simulink model "CONT_PID_CARRO"  (R2024b)
settings: Solver=VariableStepAuto  StartTime=0.0  StopTime=10.0  RelTol=1e-3
undefined symbols (not defined in the file): b_ta, K_tsa, K_tsia, T_s2
settings Model: Creator=juani  LastModifiedBy=juani

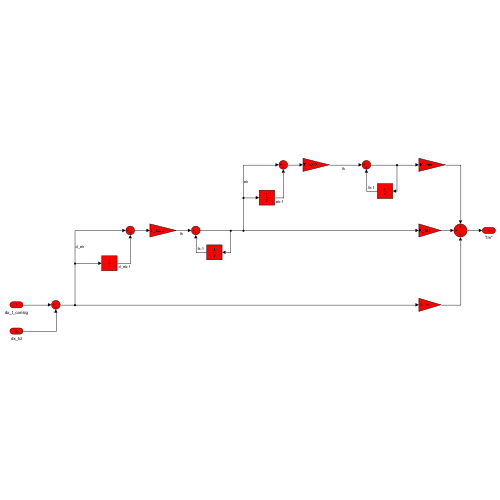
[thumbnail: Simulink's stored preview of the top-level diagram]
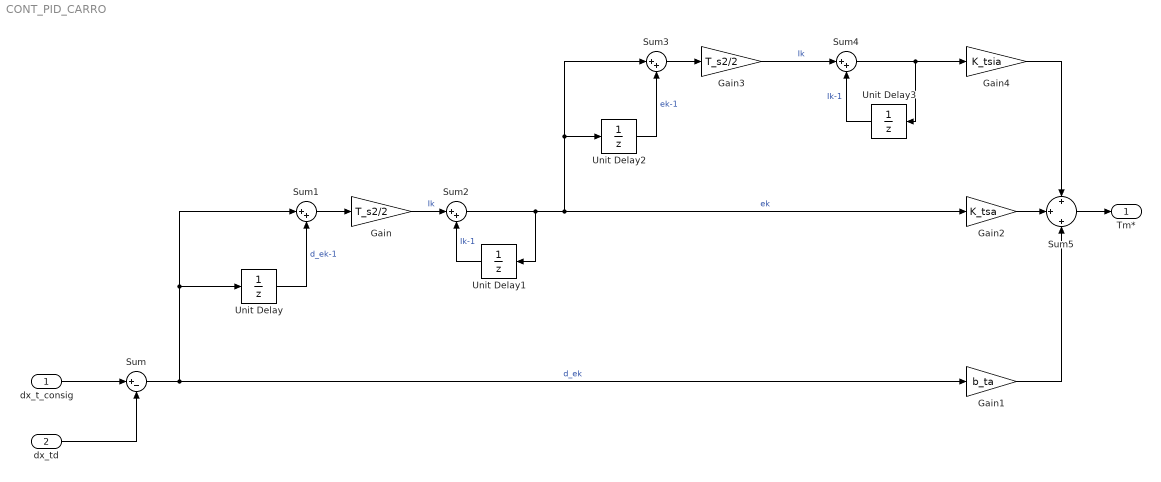
== system CONT_PID_CARRO ==
  dx_t_consig : Inport
  dx_td : Inport  Port=2
  Gain : Gain  Gain=T_s2/2
  Gain1 : Gain  Gain=b_ta
  Gain2 : Gain  Gain=K_tsa
  Gain3 : Gain  Gain=T_s2/2
  Gain4 : Gain  Gain=K_tsia
  Sum : Sum  Inputs=|+-
  Sum{1..4} (4 alike) : Sum  Inputs=|++
  Sum5 : Sum  Inputs=+|+|+
  Unit Delay{,1..3} (4 alike) : UnitDelay  SampleTime=-1  HasFrameUpgradeWarning=on
  Tm* : Outport
  wires:
  dx_td/1 -> Sum/2
  dx_t_consig/1 -> Sum/1
  Sum/1 -> Unit Delay/1, Sum1/1, Gain1/1  "d_ek"
  Unit Delay/1 -> Sum1/2  "d_ek-1"
  Sum1/1 -> Gain/1
  Gain/1 -> Sum2/1  "Ik"
  Unit Delay1/1 -> Sum2/2  "Ik-1"
  Sum2/1 -> Unit Delay1/1, Sum3/1, Unit Delay2/1, Gain2/1  "ek"
  Sum3/1 -> Gain3/1
  Unit Delay2/1 -> Sum3/2  "ek-1"
  Sum4/1 -> Unit Delay3/1, Gain4/1
  Unit Delay3/1 -> Sum4/2  "Ik-1"
  Gain3/1 -> Sum4/1  "Ik"
  Gain4/1 -> Sum5/1
  Gain2/1 -> Sum5/2
  Gain1/1 -> Sum5/3
  Sum5/1 -> Tm*/1
